simulink model "logistyczny_schemat"  (R2024b)
settings: Solver=VariableStepAuto  StartTime=0.0  StopTime=10.0  MaxStep=0.1  RelTol=1e-3
values from neighbouring files (symbols this model uses):
  K = 15    [logistyczny.m]
  N0 = [10]    [logistyczny.m]
  r = 0.1    [logistyczny.m]
settings Model: Creator=Michal  LastModifiedBy=Michal
settings DataIOCC: ReturnWorkspaceOutputs=off

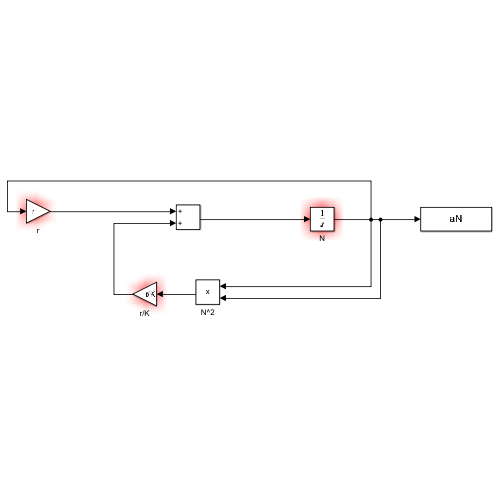
[thumbnail: Simulink's stored preview of the top-level diagram]
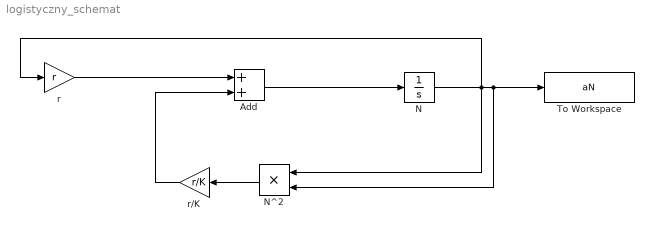
== system logistyczny_schemat ==
  Add : Sum
  N : Integrator  InitialCondition=N0
  N^2 : Product
  To Workspace : ToWorkspace  VariableName=aN  SampleTime=-1
  r : Gain  Gain=r
  r/K : Gain  Gain=r/K
  wires:
  N/1 -> N^2/1, r/1, N^2/2, To Workspace/1
  Add/1 -> N/1
  r/1 -> Add/1
  N^2/1 -> r/K/1
  r/K/1 -> Add/2
